simulink model "Oppgave2b"  (R2023a)
settings: Solver=VariableStepAuto  StartTime=0.0  StopTime=10.0  RelTol=1e-3
settings Model: Creator=augus  LastModifiedBy=augus

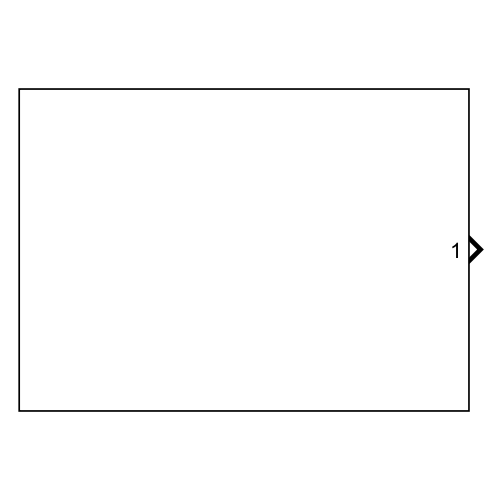
[thumbnail: Simulink's stored preview of the top-level diagram]
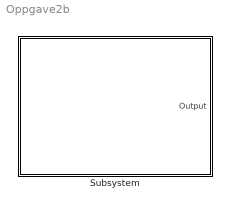
== system Oppgave2b ==
  Subsystem : Subsystem

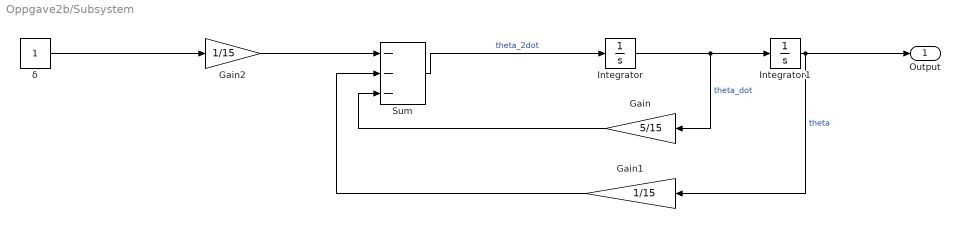
== system Oppgave2b/Subsystem ==
  Gain : Gain  Gain=5/15
  Gain1 : Gain  Gain=1/15
  Gain2 : Gain  Gain=1/15
  Integrator : Integrator
  Integrator1 : Integrator
  Sum : Sum  Inputs=---
  δ : Constant
  Output : Outport
  wires:
  Integrator1/1 -> Output/1, Gain1/1  "theta"
  Integrator/1 -> Gain/1, Integrator1/1  "theta_dot"
  Sum/1 -> Integrator/1  "theta_2dot"
  δ/1 -> Gain2/1
  Gain2/1 -> Sum/1
  Gain/1 -> Sum/3
  Gain1/1 -> Sum/2
